simulink model "simulink_Euge_apuntamiento"  (R2021a)
settings: Solver=VariableStepAuto  StartTime=0.0  StopTime=20000  FixedStep=0.001  RelTol=1e-3
undefined symbols (not defined in the file): Earth, WGS84
libraries: aerolibutil x6, sharedtransform x2, aerolib6dof2 x1, pid_lib x1, sharedutil x1, cstblocks x1
settings Model: Creator=Euge Etcheverry  LastModifiedBy=fadellavedova

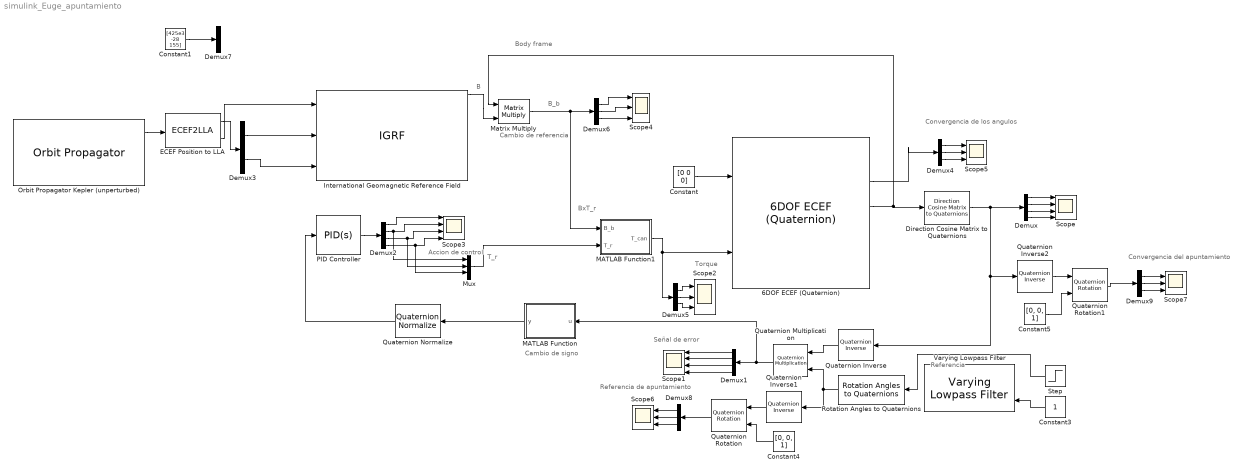
== system simulink_Euge_apuntamiento ==
  note: Convergencia del apuntamiento
  note: Referencia de apuntamiento
  note: Body frame
  note: B
  note: B_b
  note: T_r
  note: Torque
  note: Cambio de referencia
  note: BxT_r
  note: Cambio de signo
  note: Señal de error
  note: Accion de control
  note: Referencia
  note: Convergencia de los angulos
  6DOF ECEF (Quaternion) : aerolib6dof2/6DOF ECEF (Quaternion)  units=Metric (MKS)  mtype=Fixed  xg_0=[0 0 0]  Vm_0=[0 0 0]  eul_0="[0  0 0]"  pm_0=[0 0 0]  mass_0=1.0  mass_e=0.5  mass_f=2.0  inertia=2e-3*eye(3)  inertia_e=eye(3)  inertia_f=2*eye(3)  vre_flag=on  abi_flag=off  ptype=Earth (WGS84)  R=6378137  F=1/298.257223563  w_E=7292115e-11  angle_in=Internal  LG0=0  quat_statename=''  pm_statename=''  Vm_statename=''  posECEF_statename=''  posECI_statename=''  LG_statename=''  mass_statename=''
      settings: SourceProductBaseCode=AE
  Constant : Constant  Value=[0 0 0]
  Constant1 : Constant  Value=[425e3 -28 155]
  Constant3 : Constant
  Constant4 : Constant  Value=[0, 0, 1]
  Constant5 : Constant  Value=[0, 0, 1]
  Demux : Demux
  Demux1 : Demux
  Demux2 : Demux
  Demux3 : Demux  Outputs=2
  Demux{4..9} (6 alike) : Demux  Outputs=3
  Direction Cosine Matrix to Quaternions : sharedtransform/Direction Cosine Matrix  to Quaternions  aMode=0  action=None  tolerance=eps(2)
      settings: SourceProductBaseCode=AE,PW,DR,MT,UV,VE
  ECEF Position to LLA : ECEF2LLA
  International Geomagnetic Reference Field : IGRF  time_in=off  month=February  day=23  year=2024
      settings: AttributesFormatString=%<generation>
  MATLAB Function : MATLAB Function  TreatAsAtomicUnit=on
  MATLAB Function1 : MATLAB Function  TreatAsAtomicUnit=on
  Matrix Multiply : Product  Multiplication=Matrix(*)
  Mux : Mux  Inputs=3
  Orbit Propagator Kepler (unperturbed) : OrbitPropagator  startDate=[2024, 02, 23, 12, 32, 16]  eccentricity=0.0005  inclination=98.06  raan=105  trueAnomaly=180  customMu=4.305e13  customJ2=1.0826269e-03  timeFormat=Gregorian
  PID Controller : pid_lib/PID Controller  Controller=PID  Form=Parallel  TimeDomain=Continuous-time  UseExternalTs=off  SampleTime=-1  IntegratorMethod=Forward Euler  FilterMethod=Forward Euler  ControllerParametersSource=internal  P=0.1  I=0.001  D=33  UseFilter=on  N=100  TunerSelectOption=Transfer Function Based (PID Tuner App)  InitialConditionSource=internal  InitialConditionForIntegrator=0  InitialConditionForFilter=0  DifferentiatorICPrevScaledInput=0  ExternalReset=none  TrackingMode=off  Kt=1  LimitOutput=on  SatLimitsSource=internal  UpperSaturationLimit=[2e-7, 2e-7, 2e-7, 2e-7]  LowerSaturationLimit=[-2e-7, -2e-7, -2e-7, -2e-7]  LinearizeAsGain=off  AntiWindupMode=back-calculation  Kb=1  POutMin=[]  POutMax=[]  IOutMin=[]  IOutMax=[]  DOutMin=[]  DOutMax=[]  NOutMin=[]  NOutMax=[]  SumOutMin=[]  SumOutMax=[]  SaturationOutMin=[]  SaturationOutMax=[]  PParamMin=[]  PParamMax=[]  IParamMin=[]  IParamMax=[]  DParamMin=[]  DParamMax=[]  NParamMin=[]  NParamMax=[]  KbParamMin=[]  KbParamMax=[]  KtParamMin=[]  KtParamMax=[]  KbOutMin=[]  KbOutMax=[]  KtOutMin=[]  KtOutMax=[]  IntegratorOutMin=[]  IntegratorOutMax=[]  FilterOutMin=[]  FilterOutMax=[]  SumI1OutMin=[]  SumI1OutMax=[]  SumI2OutMin=[]  SumI2OutMax=[]  SumI3OutMin=[]  SumI3OutMax=[]  SumI4OutMin=[]  SumI4OutMax=[]  SumDOutMin=[]  SumDOutMax=[]  DifferentiatorOutMin=[]  DifferentiatorOutMax=[]  FilterDiffOutCoefMin=[]  FilterDiffOutCoefMax=[]  ReciprocalOutMin=[]  ReciprocalOutMax=[]  SumDenOutMin=[]  SumDenOutMax=[]  SumNumOutMin=[]  SumNumOutMax=[]  DivideOutMin=[]  DivideOutMax=[]  UdiffTsProdOutMin=[]  UdiffTsProdOutMax=[]  NTsProdOutMin=[]  NTsProdOutMax=[]  UintegralTsProdOutMin=[]  UintegralTsProdOutMax=[]  UngainTsProdOutMin=[]  UngainTsProdOutMax=[]  IntegratorContinuousStateAttributes=''  IntegratorStateMustResolveToSignalObject=off  IntegratorRTWStateStorageClass=Auto  FilterContinuousStateAttributes=''  FilterStateMustResolveToSignalObject=off  FilterRTWStateStorageClass=Auto  ParallelPVariant=InternalParameters  IdealPVariant=Disabled  IVariant=InternalParameters  DVariant=InternalParameters  IntegratorVariant=Continuous  SatVariant=Disabled  AWVariant=Passthrough  PCopyVariant=Disabled  TRVariant=Disabled  FdbkBlocksVariant=Forward  IdealPFdbkVariant=Disabled  SatFdbkVariant=Disabled  DerivativeFilterVariant=ContFilter  NVariant=InternalParameters  NCopyVariant=Disabled  FilterICVariant=InternalICsFilter  IntegratorICVariant=InternalICs  ExternalResetVariant=Disabled  TRSumVariant=Passthrough  SumFdbkVariant=Disabled  SumVariant=Sum_PID  TsampFilterVariant=InternalTs  TsampNgainVariant=Passthrough  TsampIntegralVariant=Passthrough  ExternalSaturationOutDataTypeStr=Inherit: Same as second input
  Quaternion Inverse : aerolibutil/Quaternion Inverse
  Quaternion Inverse1 : aerolibutil/Quaternion Inverse
  Quaternion Inverse2 : aerolibutil/Quaternion Inverse
  Quaternion Multiplication : aerolibutil/Quaternion Multiplication
  Quaternion Normalize : sharedutil/Quaternion Normalize  aMode=aMode
      settings: SourceProductBaseCode=AE,PW,DR,MT,UV,VE
  Quaternion Rotation : aerolibutil/Quaternion Rotation
  Quaternion Rotation1 : aerolibutil/Quaternion Rotation
  Rotation Angles to Quaternions : sharedtransform/Rotation Angles to Quaternions  rotationOrder=ZYX  aMode=aMode
      settings: SourceProductBaseCode=AE,PW,DR,MT,UV,VE
  Scope : Scope  NumInputPorts=4
  Scope1 : Scope  NumInputPorts=4
  Scope{2,4..7} (5 alike) : Scope  NumInputPorts=3
  Scope3 : Scope  NumInputPorts=4
  Step : Step  Before=[0, 0, 0]  After=[0, 0.1, 0.1]  SampleTime=0
  Varying Lowpass Filter : cstblocks/Linear Parameter Varying/Varying Lowpass Filter  N=1
  wires:
  6DOF ECEF (Quaternion)/6 -> Matrix Multiply/1, Direction Cosine Matrix to Quaternions/1
  Direction Cosine Matrix to Quaternions/1 -> Demux/1, Quaternion Inverse/1, Quaternion Inverse2/1
  Demux/1 -> Scope/1
  Demux/3 -> Scope/3
  Demux/4 -> Scope/4
  Demux/2 -> Scope/2
  Rotation Angles to Quaternions/1 -> Quaternion Inverse1/1, Quaternion Multiplication/2
  Quaternion Inverse/1 -> Quaternion Multiplication/1
  Quaternion Multiplication/1 -> MATLAB Function/1(u), Demux1/1
  Demux1/1 -> Scope1/1
  Demux1/2 -> Scope1/2
  Demux1/3 -> Scope1/3
  Demux1/4 -> Scope1/4
  PID Controller/1 -> Demux2/1
  Demux2/2 -> Mux/1, Scope3/2
  Demux2/1 -> Scope3/1
  Demux2/3 -> Mux/2, Scope3/3
  Demux2/4 -> Mux/3, Scope3/4
  Demux4/1 -> Scope5/1
  Demux4/2 -> Scope5/2
  Demux4/3 -> Scope5/3
  6DOF ECEF (Quaternion)/4 -> Demux4/1
  ECEF Position to LLA/1 -> Demux3/1
  Orbit Propagator Kepler (unperturbed)/1 -> ECEF Position to LLA/1
  International Geomagnetic Reference Field/1 -> Matrix Multiply/2
  Constant/1 -> 6DOF ECEF (Quaternion)/1
  MATLAB Function/1(y) -> Quaternion Normalize/1
  Quaternion Normalize/1 -> PID Controller/1
  Demux5/1 -> Scope2/1
  Demux5/2 -> Scope2/2
  Demux5/3 -> Scope2/3
  Demux6/1 -> Scope4/1
  Demux6/2 -> Scope4/2
  Demux6/3 -> Scope4/3
  ECEF Position to LLA/2 -> International Geomagnetic Reference Field/1
  Constant1/1 -> Demux7/1
  Demux3/1 -> International Geomagnetic Reference Field/2
  Demux3/2 -> International Geomagnetic Reference Field/3
  Matrix Multiply/1 -> MATLAB Function1/1(B_b), Demux6/1
  Constant3/1 -> Varying Lowpass Filter/2
  MATLAB Function1/1(T_can) -> 6DOF ECEF (Quaternion)/2, Demux5/1
  Mux/1 -> MATLAB Function1/2(T_r)
  Constant4/1 -> Quaternion Rotation/2
  Demux8/3 -> Scope6/3
  Demux8/2 -> Scope6/2
  Demux8/1 -> Scope6/1
  Quaternion Rotation/1 -> Demux8/1
  Quaternion Inverse1/1 -> Quaternion Rotation/1
  Demux9/3 -> Scope7/3
  Quaternion Rotation1/1 -> Demux9/1
  Constant5/1 -> Quaternion Rotation1/2
  Quaternion Inverse2/1 -> Quaternion Rotation1/1
  Demux9/2 -> Scope7/2
  Demux9/1 -> Scope7/1
  Step/1 -> Rotation Angles to Quaternions/1

== matlab function simulink_Euge_apuntamiento/MATLAB Function ==
  data: u input; y output
function y = fcn(u)
    %B_norm2 = norm(B_b)^2;
    %u_aux = u(2:4);
    %Proyecto el error sobre el plano perpendicular a B_b
    %u_proy = u_aux - (dot(u_aux, B_b)/B_norm2)*B_b;
    %u_proy = u_proy(:);
    if u(1) < 0
        y = -u; %-[u(1), u_proy'];
        y(4) = 0;
 %Ya que nuesntra planta no deberia depender de la tercer componente 
    else 
        y = u;%[u(1), u_proy'];
        y(4) = 0;
    end
end

== matlab function simulink_Euge_apuntamiento/MATLAB Function1 ==
  data: B_b input; T_can output; T_r input
function T_can = fcn(B_b, T_r)
%{
    B_escalado = B_b * 1e-9;
    B_norm = norm(B_escalado);
    if B_norm < 1e-12 %Por si es muy chico
        T_can = [0; 0; 0];
        return;
    end
    M = cross(B_escalado, T_r)/(B_norm^2);
    %Limites de saturacion del momento magnetico
    %M(3) = 0;
    M_max = 0.2;
    for i = 1:3
        if M(i) > M_max
            M(i) = M_max;
        elseif M(i) < -M_max
           M(i) = -M_max;
        end
    end
    T_can = cross(M, B_escalado);
    %}
    %T_can(3) = 0;
    %Se que T = M x B y que como queremos controlar Z, Mz = 0
    
    B = B_b * 1e-9;
    M = [0; 0; 0];
    M(1) = -T_r(2)/(B(3));
    M(2) = T_r(1)/(B(3));
    M(3) = 0;
    
    M_max = 0.2;
    for i = 1:2
        if M(i) > M_max
            M(i) = M_max;
        elseif M(i) < -M_max
            M(i) = -M_max;
        end
    end
    
    T_can = cross(M, B);
    %T_can(3) = 0;
    
    %{
    B = B_b * 1e-9;
    P = eye(3) - (B*B') / (norm(B)^2);  % Proyección ortogonal a B
    T_r = P * T_r;

    % Solo usamos Mx y My
    A = [   0      B(3);
          -B(3)     0;
           B(2)  -B(1) ];  % A @ [Mx; My] = T_can

    % Resolución de mínimos cuadrados: A * m ≈ T_r
    m = A \ T_r;

    % Saturación
    M_max = 0.2;
    m = max(min(m, M_max), -M_max);

    M = [m(1); m(2); 0];

    T_can = cross(M, B);
    %}
end
